simulink model "pitch_ap_rev"  (R2016a)
settings: Solver=FixedStepDiscrete  SolverMode=SingleTasking  StartTime=0.0  StopTime=25  FixedStep=1/40  RelTol=1e-3
model workspace (MAT data in the model file):
  dispGain = Simulink.Parameter
  dispGain.Value = 2
  dispGain.DataType = 'auto'
  dispGain.Dimensions = [1 1]
  intGain = Simulink.Parameter
  intGain.Value = 0.5
  intGain.DataType = 'auto'
  intGain.Dimensions = [1 1]
  rateGain = Simulink.Parameter
  rateGain.Value = 2
  rateGain.DataType = 'auto'
  rateGain.Dimensions = [1 1]
undefined symbols (not defined in the file): cmdLim, dispLim, intLim, rateLim
libraries: simulink x2, aerolibconvert2 x1
settings Model: ParameterArgumentNames=dispGain,intGain,rateGain  Creator=bpotter  LastModifiedBy=khouloud.gaaloul
settings DataIOCC: ExternalInput=rollIn  SaveFormat=StructureWithTime  SaveOutput=off  DSMLogging=off  SaveTime=off  OutputSaveName=Ail_Cmd  SignalLoggingName=pitch_ap_logsout
settings OptimizationCC: BlockReduction=off  DefaultParameterBehavior=Inlined  InlineInvariantSignals=on  EnhancedBackFolding=on  ExpressionDepthLimit=2147483647  EfficientFloat2IntCast=on  EfficientMapNaN2IntZero=off  OptimizeModelRefInitCode=on  MaxStackSize=inf
settings DebuggingCC: SignalInfNanChecking=error  SignalRangeChecking=error  ReadBeforeWriteMsg=EnableAllAsError  WriteAfterWriteMsg=EnableAllAsError  WriteAfterReadMsg=EnableAllAsError  AlgebraicLoopMsg=error  ArtificialAlgebraicLoopMsg=error  SaveWithDisabledLinksMsg=error  SaveWithParameterizedLinksMsg=error  CheckExecutionContextPreStartOutputMsg=on  CheckExecutionContextRuntimeOutputMsg=on  BlockPriorityViolationMsg=error  MaxConsecutiveZCsMsg=warning  SolverPrmCheckMsg=error  InheritedTsInSrcMsg=error  SingleTaskRateTransMsg=error  TasksWithSamePriorityMsg=error  SigSpecEnsureSampleTimeMsg=error  CheckMatrixSingularityMsg=error  IntegerOverflowMsg=error  ParameterUnderflowMsg=error  ParameterPrecisionLossMsg=error  ParameterTunabilityLossMsg=error  UnderSpecifiedDataTypeMsg=error  UnnecessaryDatatypeConvMsg=warning  VectorMatrixConversionMsg=error  SignalLabelMismatchMsg=error  UnconnectedInputMsg=error  UnconnectedOutputMsg=error  UnconnectedLineMsg=error  SFcnCompatibilityMsg=error  UniqueDataStoreMsg=error  BusObjectLabelMismatch=error  RootOutportRequireBusObject=error  AssertControl=DisableAll  ModelReferenceIOMsg=error  ModelReferenceIOMismatchMessage=error  UnknownTsInhSupMsg=error  ModelReferenceDataLoggingMessage=error  ModelReferenceExtraNoncontSigs=none  StateNameClashWarn=warning  StrictBusMsg=ErrorOnBusTreatedAsVector  NonBusSignalsTreatedAsBus=error  IntegerSaturationMsg=error
settings HardwareCC: ProdBitPerPointer=32  ProdLargestAtomicFloat=None  ProdEndianess=BigEndian  ProdWordSize=32  ProdHWDeviceType=32-bit Embedded Processor  TargetHWDeviceType=32-bit Generic
settings ModelReferenceCC: PropagateSignalLabelsOutOfModel=off
settings RTWCC: SystemTargetFile=ert.tlc  TemplateMakefile=ert_default_tmf  GenerateReport=on  RTWVerbose=off  IncludeHyperlinkInReport=on  LaunchReport=on  PortableWordSizes=on  GenerateTraceInfo=on  GenerateTraceReport=on  GenerateTraceReportSl=on  GenerateTraceReportSf=on  GenerateTraceReportEml=on
settings CodeAppCC: ForceParamTrailComments=on  IgnoreCustomStorageClasses=off  MaxIdLength=63  MangleLength=4  CustomSymbolStrType=$N$R$M  InternalIdentifier=Classic  ReqsInCode=on
settings ERTTargetCC: UtilityFuncGeneration=Shared location  IncludeMdlTerminateFcn=off  GeneratePreprocessorConditionals=Disable all  SuppressErrorStatus=on  SupportAbsoluteTime=off  SupportNonFinite=off  SupportComplex=off  ParenthesesLevel=Maximum  InlinedParameterPlacement=NonHierarchical  ERTCustomFileTemplate=example_file_process.tlc  PreserveExpressionOrder=on  PreserveIfCondition=on  ConvertIfToSwitch=off  SuppressUnreachableDefaultCases=off
settings ConfigComp: CovSaveName=covdata_pitchAP  CovMetricSettings=dcmtrzoie  CovHTMLOptions=-sRT=1 -aTS=1 -bRG=1 -bTC=1 -hTR=1 -nFC=0 -scm=1 -bcm=1 -xEv=0  CovHtmlReporting=off  CovSaveSingleToWorkspaceVar=off  CovCumulativeVarName=covCumulativeData_pitchAP  CovCumulativeReport=on  CovReportOnPause=off  CovModelRefEnable=Off

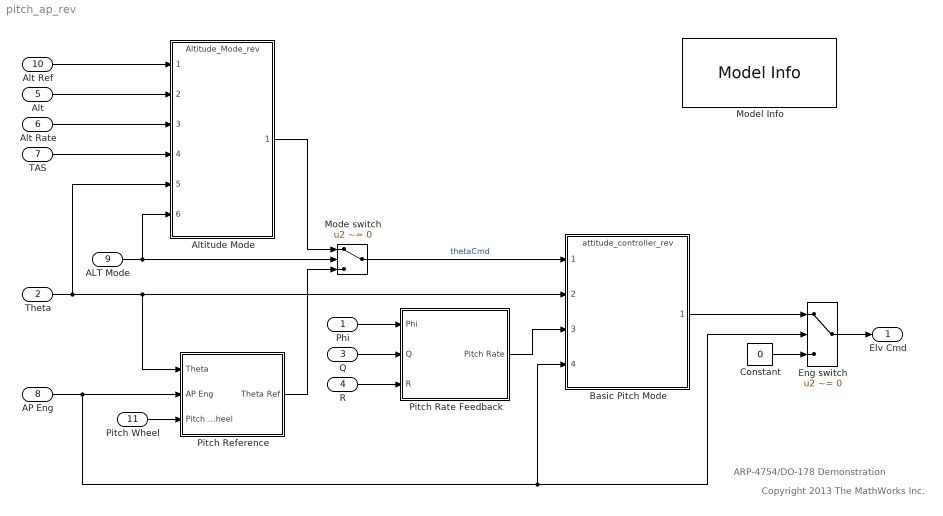
== system pitch_ap_rev ==
  note: Copyright 2013 The MathWorks Inc.
  note: ARP-4754/DO-178 Demonstration
  Phi : Inport  OutDataTypeStr=double  PortDimensions=1  SampleTime=1/40  Interpolate=off
  Theta : Inport  Port=2  OutDataTypeStr=double  PortDimensions=1  SampleTime=1/40  Interpolate=off
  Q : Inport  Port=3  OutDataTypeStr=double  PortDimensions=1  SampleTime=1/40  Interpolate=off
  R : Inport  Port=4  OutDataTypeStr=double  PortDimensions=1  SampleTime=1/40  Interpolate=off
  Alt : Inport  Port=5  OutDataTypeStr=double  PortDimensions=1  SampleTime=1/40  Interpolate=off
  Alt Rate : Inport  Port=6  OutDataTypeStr=double  PortDimensions=1  SampleTime=1/40  Interpolate=off
  TAS : Inport  Port=7  OutDataTypeStr=double  PortDimensions=1  SampleTime=1/40  Interpolate=off
  AP Eng : Inport  Port=8  OutDataTypeStr=boolean  PortDimensions=1  SampleTime=1/40  Interpolate=off
  ALT Mode : Inport  Port=9  OutDataTypeStr=boolean  PortDimensions=1  SampleTime=1/40  Interpolate=off
  Alt Ref : Inport  Port=10  OutDataTypeStr=double  PortDimensions=1  SampleTime=1/40  Interpolate=off
  "Pitch Wheel " : Inport  Port=11  OutDataTypeStr=double  PortDimensions=1  SampleTime=1/40  Interpolate=off
  Altitude Mode : ModelReference  ModelNameDialog=Altitude_Mode_rev  SimulationMode=Normal  ModelReferenceVersion=1.100
  Basic Pitch Mode : ModelReference  RequirementInfo={} %GIDa_a8a1316c_a2d9_4453_bd2a_6f526e87d6f7  ModelNameDialog=attitude_controller_rev  ParameterArgumentNames=dispGain,dispLim,rateGain,rateLim,intGain,intLim,cmdLim  ParameterArgumentValues=dispGain,20,rateGain,3,intGain,5,20  SimulationMode=Normal  ModelReferenceVersion=1.70
  Constant : Constant  Value=0  OutDataTypeStr=double
  Eng switch : Switch  Criteria=u2 ~= 0
  Mode switch : Switch  Criteria=u2 ~= 0
  Model Info : simulink/Model-Wide Utilities/Model Info  BlockCM=None  Frame=on  DisplayStringWithTags=|  HorizontalTextAlignment=Left  LeftAlignmentValue=0.02  SourceBlockDiagram=pitch_ap_rev  TagMaxNumber=20
      | Pitch Autopilot
      | Author: %<LastModifiedBy>
      | Date: %<LastModificationDate>
      | Model Version: %<ModelVersion>
  Pitch Rate Feedback : Subsystem  TreatAsAtomicUnit=on
      settings: RTWSystemCode=Inline
  Pitch Reference : Subsystem  TreatAsAtomicUnit=on
      settings: RTWSystemCode=Inline
  Elv Cmd : Outport  OutDataTypeStr=double  PortDimensions=1  SampleTime=1/40
  wires:
  Alt Ref/1 -> Altitude Mode/1
  Theta/1 -> Pitch Reference/1(Theta), Basic Pitch Mode/2, Altitude Mode/5
  Q/1 -> Pitch Rate Feedback/2(Q)
  Alt/1 -> Altitude Mode/2
  Alt Rate/1 -> Altitude Mode/3
  Mode switch/1 -> Basic Pitch Mode/1  "thetaCmd"
  ALT Mode/1 -> Mode switch/2, Altitude Mode/6
  Altitude Mode/1 -> Mode switch/1
  AP Eng/1 -> Eng switch/2, Basic Pitch Mode/4, Pitch Reference/2(AP Eng)
  Eng switch/1 -> Elv Cmd/1
  Constant/1 -> Eng switch/3
  Phi/1 -> Pitch Rate Feedback/1(Phi)
  R/1 -> Pitch Rate Feedback/3(R)
  TAS/1 -> Altitude Mode/4
  Pitch Reference/1(Theta Ref) -> Mode switch/3
  "Pitch Wheel "/1 -> Pitch Reference/3(Pitch Wheel)
  Pitch Rate Feedback/1(Pitch Rate) -> Basic Pitch Mode/3
  Basic Pitch Mode/1 -> Eng switch/1

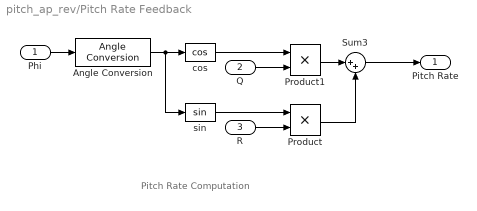
== system pitch_ap_rev/Pitch Rate Feedback ==
  note: Pitch Rate Computation
  Phi : Inport
  Q : Inport  Port=2
  R : Inport  Port=3
  Angle Conversion : aerolibconvert2/Angle Conversion  IU=deg  OU=rad
  Product : Product  RndMeth=Zero
  Product1 : Product  RndMeth=Zero
  Sum3 : Sum  Inputs=|++
  cos : Trigonometry  Operator=cos  OutputSignalType=real
  sin : Trigonometry  OutputSignalType=real
  Pitch Rate : Outport
  wires:
  Phi/1 -> Angle Conversion/1
  Product/1 -> Sum3/2
  sin/1 -> Product/1
  R/1 -> Product/2
  Angle Conversion/1 -> sin/1, cos/1
  Product1/1 -> Sum3/1
  cos/1 -> Product1/1
  Q/1 -> Product1/2
  Sum3/1 -> Pitch Rate/1

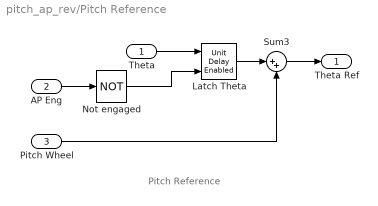
== system pitch_ap_rev/Pitch Reference ==
  note: Pitch Reference
  Theta : Inport
  AP Eng : Inport  Port=2
  Pitch Wheel : Inport  Port=3
  Latch Theta : simulink/Additional Math & Discrete/Additional Discrete/Unit Delay Enabled  vinit=0.0  tsamp=1/40
  Not engaged : Logic  Operator=NOT  IconShape=distinctive  AllPortsSameDT=off  OutDataTypeStr=boolean
  Sum3 : Sum  Inputs=|++
  Theta Ref : Outport
  wires:
  Not engaged/1 -> Latch Theta/2
  Latch Theta/1 -> Sum3/1
  Theta/1 -> Latch Theta/1
  AP Eng/1 -> Not engaged/1
  Sum3/1 -> Theta Ref/1
  Pitch Wheel/1 -> Sum3/2
